simulink model "ExtendedKalmanFilter"  (R2024b)
settings: Solver=VariableStepAuto  StartTime=0.0  StopTime=20  RelTol=1e-3
undefined symbols (not defined in the file or in its folder): A, B, C, Continuous, Time, Ts
libraries: simulink x2, sharedTrackingLibrary x1, ctrlSharedLib x1
settings Model: Creator=felixzauner  LastModifiedBy=felixzauner

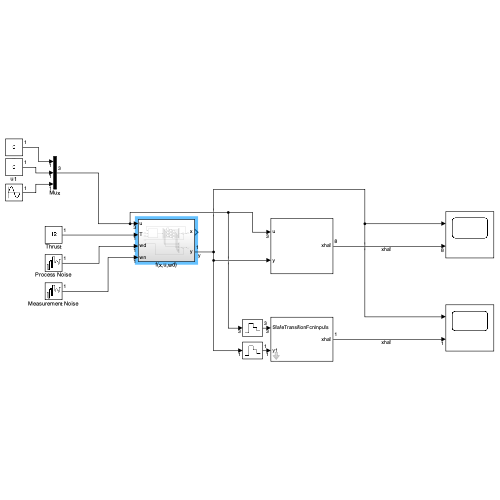
[thumbnail: Simulink's stored preview of the top-level diagram]
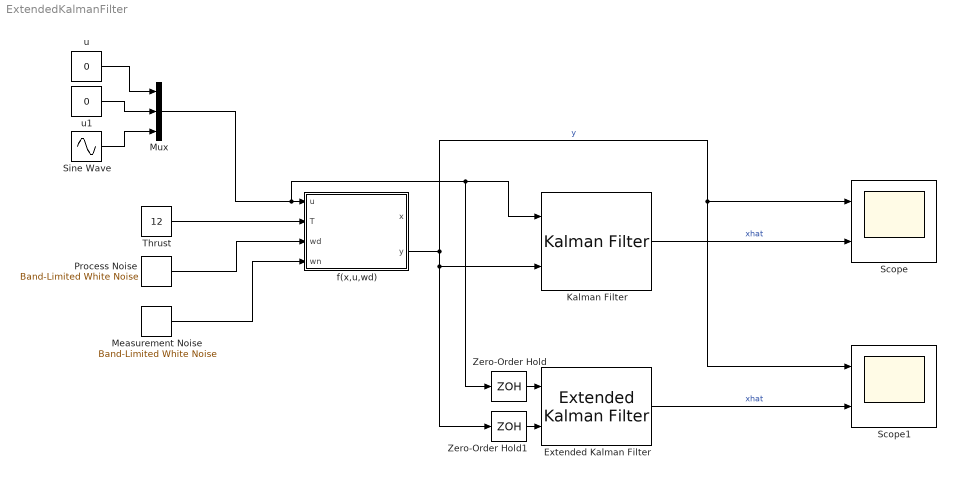
== system ExtendedKalmanFilter ==
  Extended Kalman Filter : sharedTrackingLibrary/Extended Kalman Filter  StateTransitionFcn=myStateTransitionFcn  HasStateTransitionJacobianFcn=off  HasAdditiveProcessNoise=Additive  ProcessNoise=1  HasTimeVaryingProcessNoise=off  HasStateTransitionFcnExtraArgument=1  InitialState=0  InitialStateCovariance=1  MeasurementFcn1=myMeasurementFcn  HasMeasurementJacobianFcn1=off  HasMeasurementEnablePort1=off  HasAdditiveMeasurementNoise1=Additive  MeasurementNoise1=1  HasTimeVaryingMeasurementNoise1=off  HasMeasurementFcnExtraArgument1=0  HasMeasurementWrapping1=off  MeasurementFcn2=myMeasurementFcn  HasMeasurementJacobianFcn2=off  HasMeasurementEnablePort2=off  HasAdditiveMeasurementNoise2=Additive  MeasurementNoise2=1  HasTimeVaryingMeasurementNoise2=off  HasMeasurementFcnExtraArgument2=0  HasMeasurementWrapping2=off  MeasurementFcn3=myMeasurementFcn  HasMeasurementJacobianFcn3=off  HasMeasurementEnablePort3=off  HasAdditiveMeasurementNoise3=Additive  MeasurementNoise3=1  HasTimeVaryingMeasurementNoise3=off  HasMeasurementFcnExtraArgument3=0  HasMeasurementWrapping3=off  MeasurementFcn4=myMeasurementFcn  HasMeasurementJacobianFcn4=off  HasMeasurementEnablePort4=off  HasAdditiveMeasurementNoise4=Additive  MeasurementNoise4=1  HasTimeVaryingMeasurementNoise4=off  HasMeasurementFcnExtraArgument4=0  HasMeasurementWrapping4=off  MeasurementFcn5=myMeasurementFcn  HasMeasurementJacobianFcn5=off  HasMeasurementEnablePort5=off  HasAdditiveMeasurementNoise5=Additive  MeasurementNoise5=1  HasTimeVaryingMeasurementNoise5=off  HasMeasurementFcnExtraArgument5=0  HasMeasurementWrapping5=off  EnableMultirate=off  StateTransitionFcnSampleTime=1  MeasurementFcn1SampleTime=1  MeasurementFcn2SampleTime=1  MeasurementFcn3SampleTime=1  MeasurementFcn4SampleTime=1  MeasurementFcn5SampleTime=1  UseCurrentEstimator=on  OutputStateCovariance=off  DataType=double  SampleTime=Ts  NumberOfMeasurements=1
  Kalman Filter : ctrlSharedLib/Kalman Filter  TimeDomain=Continuous-Time  UseCurrentEstimator=on  ModelSource=Individual A, B, C, D matrices  ModelSourceVariable=ss(0.95,1,1,0,1)  A=A  B=B  C=C  D=0  NumberOfStates=1  NumberOfInputs=1  NumberOfOutputs=1  InitialEstimateSource=Dialog  X0=[0 0 0 0 0 0 0 0]  P0=10  UseK=off  UseGH=off  NumberOfProcessNoiseInputs=1  G=1  TimeInvariantG=on  H=0  TimeInvariantH=on  Q=Q  TimeInvariantQ=on  R=1  TimeInvariantR=on  N=0  TimeInvariantN=on  AddInputPort=on  AddEnablePort=off  OutputEstimatedY=off  OutputP=off  Ts=-1
  Measurement Noise : simulink/Sources/Band-Limited White Noise  Cov=Ts  Ts=Ts  seed=[1423]
  Mux : Mux  Inputs=3
  Process Noise : simulink/Sources/Band-Limited White Noise  Cov=0  Ts=Ts  seed=[23341]
  Scope : Scope  NumInputPorts=2
  Scope1 : Scope  NumInputPorts=2
  Sine Wave : Sin  Amplitude=0.1  SampleTime=0
  Thrust : Constant  Value=12
  Zero-Order Hold : ZeroOrderHold  SampleTime=Ts
  Zero-Order Hold1 : ZeroOrderHold  SampleTime=Ts
  f(x,u,wd) : Subsystem
  u : Constant  Value=0
  u1 : Constant  Value=0
  wires:
  f(x,u,wd)/2(y) -> Zero-Order Hold1/1, Kalman Filter/2, Scope/1, Scope1/1  "y"
  Kalman Filter/1 -> Scope/2  "xhat"
  Thrust/1 -> f(x,u,wd)/2(T)
  Process Noise/1 -> f(x,u,wd)/3(wd)
  Measurement Noise/1 -> f(x,u,wd)/4(wn)
  u/1 -> Mux/1
  u1/1 -> Mux/2
  Sine Wave/1 -> Mux/3
  Mux/1 -> Kalman Filter/1, Zero-Order Hold/1, f(x,u,wd)/1(u)
  Extended Kalman Filter/1 -> Scope1/2  "xhat"
  Zero-Order Hold/1 -> Extended Kalman Filter/1
  Zero-Order Hold1/1 -> Extended Kalman Filter/2

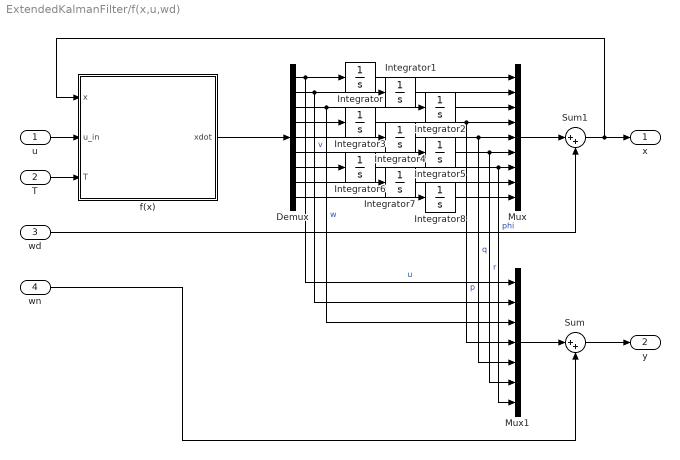
== system ExtendedKalmanFilter/f(x,u,wd) ==
  u : Inport
  T : Inport  Port=2
  wd : Inport  Port=3
  wn : Inport  Port=4
  Demux : Demux  Outputs=9
  Integrator : Integrator  InitialCondition=20
  Integrator{1..8} (8 alike) : Integrator
  Mux : Mux  Inputs=9
  Mux1 : Mux  Inputs=7
  Sum : Sum  Inputs=|++
  Sum1 : Sum  Inputs=|++
  f(x) : MATLAB Function  TreatAsAtomicUnit=on
  x : Outport
  y : Outport  Port=2
  wires:
  u/1 -> f(x)/2(u_in)
  Demux/1 -> Mux1/1, Integrator/1  "u"
  Demux/2 -> Integrator1/1, Mux1/2  "v"
  Demux/3 -> Mux1/3, Integrator2/1  "w"
  Demux/4 -> Integrator3/1
  Demux/5 -> Integrator4/1
  Demux/6 -> Integrator5/1
  Demux/7 -> Integrator6/1
  Demux/8 -> Integrator7/1
  Demux/9 -> Integrator8/1
  Integrator2/1 -> Mux/3
  Integrator5/1 -> Mux/6, Mux1/6  "r"
  Integrator8/1 -> Mux/9
  Integrator1/1 -> Mux/2
  Integrator3/1 -> Mux/4, Mux1/4  "p"
  Integrator4/1 -> Mux/5, Mux1/5  "q"
  Integrator6/1 -> Mux1/7, Mux/7  "phi"
  Integrator7/1 -> Mux/8
  T/1 -> f(x)/3(T)
  Integrator/1 -> Mux/1
  Mux1/1 -> Sum/1
  Sum/1 -> y/1
  wn/1 -> Sum/2
  f(x)/1(xdot) -> Demux/1
  wd/1 -> Sum1/2
  Mux/1 -> Sum1/1
  Sum1/1 -> f(x)/1(x), x/1

== matlab function ExtendedKalmanFilter/f(x,u,wd)/f(x) ==
  data: x input; xdot output; u_in input; T input
% Nonlinear Function for a Rocket
function xdot = rocket_f(x, u_in,T)
% x = [u v w p q r phi theta psi]'
% u_in = [delta_eta delta_zeta delta_r T]' 

% Define Parameters
% --- Geometry / environment ---
g0   = 9.81;        % m/s^2
rho0 = 1.225;       % kg/m^3 (sea level)
S    = 0.010;       % m^2  reference area
d    = 0.10;        % m    reference diameter

% --- Mass / inertia ---
m  = 1.20;          % kg
Ix = 0.005;         % kg*m^2
Iy = 0.020;         % kg*m^2 
Iz = 0.020;         % kg*m^2

% --- Aerodynamic force coeffs ---
CA0       = 0.09;   % axial (drag-like)
CA_kalpha = 0.041;   % axial vs alpha
CA_kbeta  = 0.041;   % axial vs beta


% --- Moment coeffs ---
Cl_delta = 0.229;    % roll control effectiveness
Clp      = -10;     % roll damping
Cm_alpha = 2.0;    % pitch stability derivative
Cm_delta = 1.432;    % pitch control effectiveness
Cmq      = -10;     % pitch damping
Cn_beta  = 2.0;     % yaw stability derivative
Cn_delta = 1.432;     % yaw control effectiveness
Cnr      = -10;     % yaw damping

CN_alpha = -10;
CN_delta = -0.1;

% --- Reference points ---
xcm  = 0.50;        % m 
xref = 0.45;        % m 

% --- unpack state ---
ub    = x(1);  vb = x(2);  wb = x(3);       
p     = x(4);  q  = x(5);  r  = x(6);
phi   = x(7);  theta = x(8); psi = x(9);

% --- unpack inputs ---
delta_eta  = u_in(1);
delta_zeta = u_in(2);
delta_r    = u_in(3);


% --- derived quantities ---
V = sqrt(ub^2 + vb^2 + wb^2) + 1e-9;  % avoid div0
alpha = atan2(wb,ub);
beta  = asin(vb / V); 
alpha_total = atan2(sqrt(vb^2 + wb^2), ub);
% Dynamic pressure q = 1/2 p V^2 for moments
Qdyn = 0.5*rho0*V^2;


CA = CA0 + CA_kalpha*alpha + CA_kbeta*beta;
CN = CN_alpha * alpha_total; %+ CN_delta * delta_eff;
% Build direct force coefficiants
CNy = CN * vb / sqrt(vb^2 + wb^2 + 1e-9);
CNz = CN * wb / sqrt(vb^2 + wb^2 + 1e-9);

% Aerodynamic forces 
FAxb = -Qdyn * CA  * S;
FAyb =  Qdyn * CNy * S;
FAzb =  Qdyn * CNz * S;

% --- thrust in body ---
FPxb = T;  FPyb = 0;  FPzb = 0;

% --- gravity in body: Fg_b = R_nb' * [0;0;mg] in NED ---
% NED: gravity in nav frame is [0;0; +m*g] (Down positive)
Fg_n = [-m*g0; 0;0];

% Rotation matrix R_b^n (ZYX) and R_n^b = (R_b^n)'
cphi = cos(phi); sphi = sin(phi);
cth  = cos(theta); sth = sin(theta);
cps  = cos(psi); sps  = sin(psi);

% ZYX: body->nav (matches common aerospace convention)
R_b_n = [ cth*cps,  sphi*sth*cps - cphi*sps,  cphi*sth*cps + sphi*sps;
          cth*sps,  sphi*sth*sps + cphi*cps,  cphi*sth*sps - sphi*cps;
          -sth,     sphi*cth,              cphi*cth ];
R_n_b = R_b_n';

Fg_b = R_n_b * Fg_n;
Fgxb = Fg_b(1); Fgyb = Fg_b(2); Fgzb = Fg_b(3);

% --- total forces ---
Fx = FAxb + FPxb + Fgxb;
Fy = FAyb + FPyb + Fgyb;
Fz = FAzb + FPzb + Fgzb;

% --- moment coefficients  ---
Cl = Cl_delta*delta_r + (d/(2*V))*Clp*p;

% Pitch & yaw moment coefficients
Cmref = Cm_alpha*alpha + Cm_delta*delta_eta;
Cnref = Cn_beta *beta  + Cn_delta*delta_zeta;

Cm = Cmref - CNz*((xcm-xref)/d) + (d/(2*V))*(Cmq + Cm_alpha)*q;
Cn = Cnref - CNy*((xcm-xref)/d) + (d/(2*V))*(Cnr + Cn_beta )*r;

LA = Qdyn * Cl * S * d;
MA = Qdyn * Cm * S * d;
NA = Qdyn * Cn * S * d;

% Propulsion moments 
Lp = 0; Mp = 0; Np = 0;

% --- translational dynamics in body ---
udot = Fx/m - (q*wb - r*vb);
vdot = Fy/m - (r*ub - p*wb);
wdot = Fz/m - (p*vb - q*ub);

% --- rotational dynamics ---
pdot = (LA + Lp - q*r*(Iz - Iy))/Ix;
qdot = (MA + Mp - r*p*(Ix - Iz))/Iy;
rdot = (NA + Np - p*q*(Iy - Ix))/Iz;

% --- Euler kinematics ---
phidot   = p + (q*sin(phi) + r*cos(phi))*tan(theta);
thetadot = q*cos(phi) - r*sin(phi);
psidot   = (q*sin(phi) + r*cos(phi))/cos(theta);

xdot = [udot vdot wdot pdot qdot rdot phidot thetadot psidot];
end
